simulink model "accelerate"  (R2022a)
settings: Solver=FixedStepDiscrete  StartTime=0.0  StopTime=inf  RelTol=1e-3  EnableMultiTasking=on
InitFcn:
  | run('busObjects.m')
model workspace (MAT data in the model file):
  omega = 8
  zeta = 0.05
undefined symbols (not defined in the file or in its folder): HS, IO291
libraries: aru_toolbox x6, eeGeneralControl x4, speedgoatlib_IO691 x3, speedgoatlib_IO291 x1
settings Model: SimulationMode=external  Creator=Mechatronics  LastModifiedBy=Mechatronics
settings SolverCC: ConcurrentTasks=on  AlgebraicLoopSolver=TrustRegion  PositivePriorityOrder=on  InsertRTBMode=Never (minimum delay)
settings DataIOCC: SaveFormat=Array  SaveState=on  SignalLoggingName=logsOut
settings OptimizationCC: BlockReduction=off  BooleanDataType=off  OptimizeBlockIOStorage=off  BufferReuse=off  GlobalBufferReuse=off  ExpressionFolding=off  LocalBlockOutputs=off  InitFltsAndDblsToZero=on  OptimizeDataStoreBuffers=off  BusAssignmentInplaceUpdate=off
settings DebuggingCC: SaveWithParameterizedLinksMsg=none  UnderspecifiedInitializationDetection=Classic  MergeDetectMultiDrivingBlocksExec=none  CheckExecutionContextPreStartOutputMsg=on  SignalResolutionControl=TryResolveAllWithWarning  TasksWithSamePriorityMsg=none  UnconnectedInputMsg=warning  UnconnectedOutputMsg=warning  UnconnectedLineMsg=warning  SFUnexpectedBacktrackingDiag=warning  SFNoUnconditionalDefaultTransitionDiag=warning  SFExecutionAtInitializationDiag=none  SFMachineParentedDataDiag=warning  ArithmeticOperatorsInVariantConditions=warning
settings HardwareCC: ProdBitPerLong=64  ProdLongLongMode=on  ProdHWDeviceType=Intel->x86-64 (Linux 64)
settings ModelReferenceCC: PropagateSignalLabelsOutOfModel=off
settings SFSimCC: SimUseLocalCustomCode=off  SimTargetLang=C++
settings RTWCC: Description=Simulink Real-Time  SystemTargetFile=slrealtime.tlc  TemplateMakefile=slrealtime_default_tmf  RTWUseLocalCustomCode=off  Toolchain=Simulink Real-Time Toolchain  BuildConfiguration=Faster Runs  CodeExecutionProfiling=on  TargetLang=C++  DLArmComputeVersion=19.05
settings CodeAppCC: StateflowObjectComments=on
settings SimulinkRealTimeTargetCC: MATLABClassNameForMDSCustomization=Simulink.SoftwareTarget.GRTCustomization  UseGCCFastMath=on
settings ConfigComp: CovMetricSettings=dw  CovSaveCumulativeToWorkspaceVar=on  CovSaveSingleToWorkspaceVar=on  CovExternalEMLEnable=off  CovSFcnEnable=off

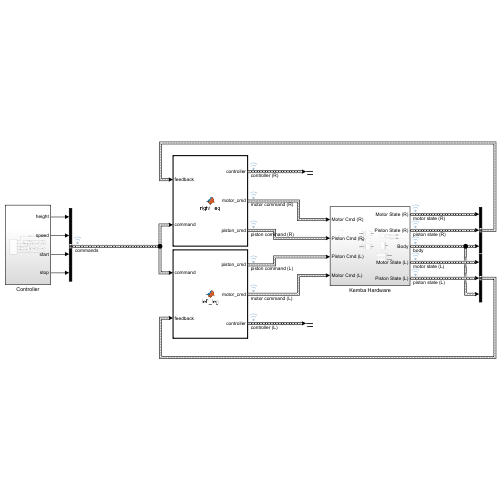
[thumbnail: Simulink's stored preview of the top-level diagram]
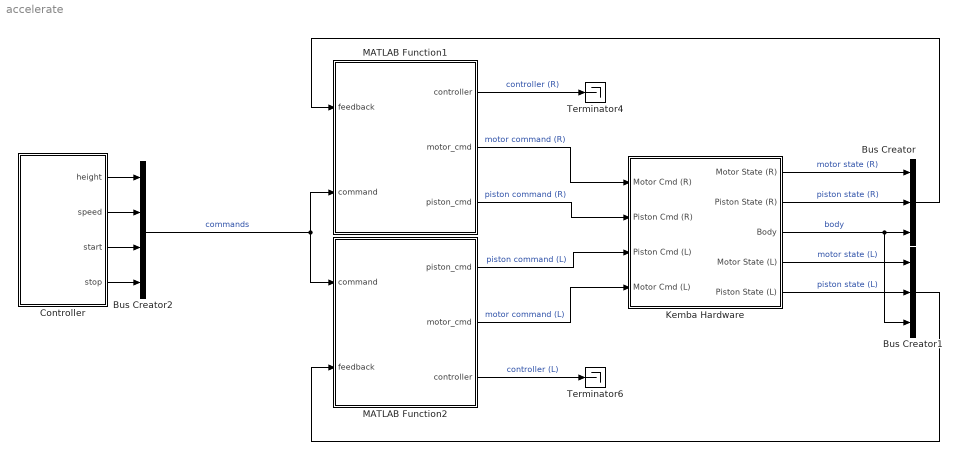
== system accelerate ==
  Bus Creator : BusCreator  Inputs=3  OutDataTypeStr=Bus: State  NonVirtualBus=on
      settings: InheritFromInputs=off
  Bus Creator1 : BusCreator  Inputs=3  OutDataTypeStr=Bus: State  NonVirtualBus=on
      settings: InheritFromInputs=off
  Bus Creator2 : BusCreator  Inputs=4  OutDataTypeStr=Bus: Command  NonVirtualBus=on
      settings: InheritFromInputs=off
  Controller : Subsystem
  Kemba Hardware : Subsystem
  MATLAB Function1 : MATLAB Function  TreatAsAtomicUnit=on  SystemSampleTime=0.001
  MATLAB Function2 : MATLAB Function  TreatAsAtomicUnit=on  SystemSampleTime=0.001
  Terminator4 : Terminator
  Terminator6 : Terminator
  wires:
  MATLAB Function1/3(piston_cmd) -> Kemba Hardware/2(Piston Cmd (R))  "piston command (R)"
  MATLAB Function2/1(piston_cmd) -> Kemba Hardware/3(Piston Cmd (L))  "piston command (L)"
  MATLAB Function1/2(motor_cmd) -> Kemba Hardware/1(Motor Cmd (R))  "motor command (R)"
  MATLAB Function2/2(motor_cmd) -> Kemba Hardware/4(Motor Cmd (L))  "motor command (L)"
  Kemba Hardware/4(Motor State (L)) -> Bus Creator1/1  "motor state (L)"
  Kemba Hardware/5(Piston State (L)) -> Bus Creator1/2  "piston state (L)"
  Kemba Hardware/3(Body) -> Bus Creator1/3, Bus Creator/3  "body"
  Kemba Hardware/2(Piston State (R)) -> Bus Creator/2  "piston state (R)"
  Kemba Hardware/1(Motor State (R)) -> Bus Creator/1  "motor state (R)"
  Bus Creator/1 -> MATLAB Function1/1(feedback)
  Bus Creator1/1 -> MATLAB Function2/2(feedback)
  Bus Creator2/1 -> MATLAB Function2/1(command), MATLAB Function1/2(command)  "commands"
  Controller/2(speed) -> Bus Creator2/2
  MATLAB Function1/1(controller) -> Terminator4/1  "controller (R)"
  MATLAB Function2/3(controller) -> Terminator6/1  "controller (L)"
  Controller/1(height) -> Bus Creator2/1
  Controller/3(start) -> Bus Creator2/3
  Controller/4(stop) -> Bus Creator2/4

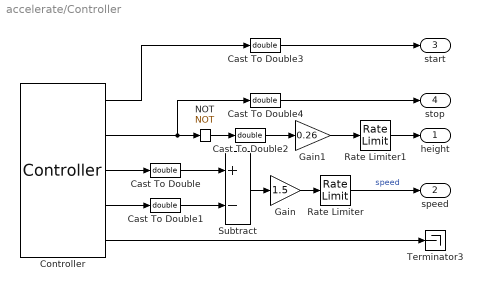
== system accelerate/Controller ==
  Cast To Double{,1..4} (5 alike) : DataTypeConversion  OutDataTypeStr=double  SaturateOnIntegerOverflow=off  RndMeth=Floor
  Controller : aru_toolbox/Controller
      link override "LVTTL digital input ": parInternalModuleId=1
      settings: SourceProductName=ARU Toolbox
  Gain : Gain  Gain=1.5
  Gain1 : Gain  Gain=0.26
  NOT : Logic  Operator=NOT  IconShape=distinctive  AllPortsSameDT=off  OutDataTypeStr=boolean
  Rate Limiter : RateLimiter  RisingSlewLimit=0.3  FallingSlewLimit=-0.3  SampleTimeMode=inherited
  Rate Limiter1 : RateLimiter  RisingSlewLimit=0.05  FallingSlewLimit=-0.05  SampleTimeMode=inherited  InitialCondition=0.26
  Subtract : Sum  Inputs=+-
  Terminator3 : Terminator
  height : Outport
  speed : Outport  Port=2
  start : Outport  Port=3
  stop : Outport  Port=4
  wires:
  Gain1/1 -> Rate Limiter1/1
  Rate Limiter/1 -> speed/1  "speed"
  Subtract/1 -> Gain/1
  Controller/5 -> Terminator3/1
  Controller/2 -> Cast To Double4/1, NOT/1
  Controller/3 -> Cast To Double/1
  Gain/1 -> Rate Limiter/1
  Controller/4 -> Cast To Double1/1
  Cast To Double/1 -> Subtract/1
  Cast To Double1/1 -> Subtract/2
  Controller/1 -> Cast To Double3/1
  Rate Limiter1/1 -> height/1
  Cast To Double3/1 -> start/1
  NOT/1 -> Cast To Double2/1
  Cast To Double2/1 -> Gain1/1
  Cast To Double4/1 -> stop/1

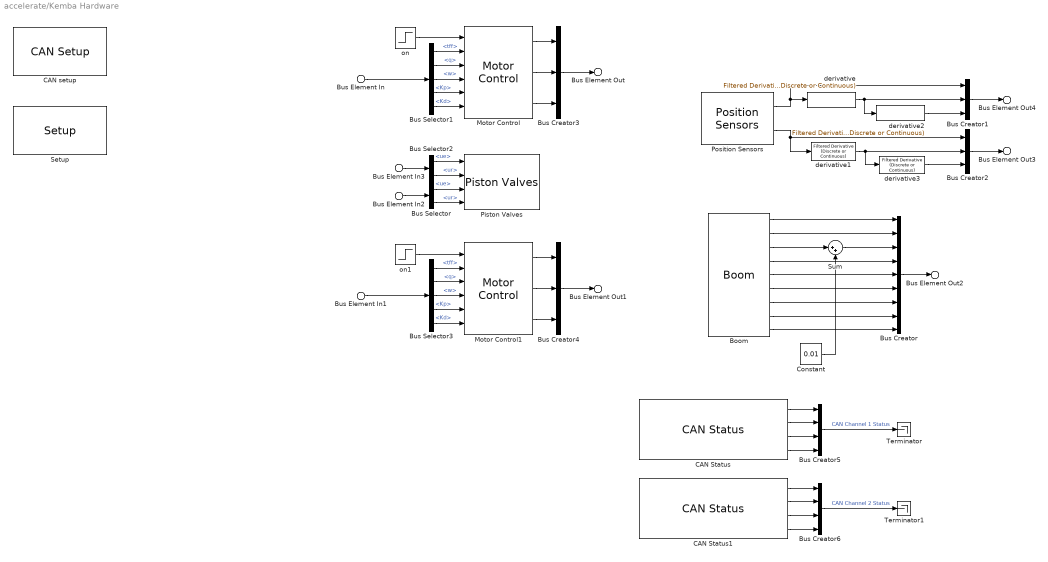
== system accelerate/Kemba Hardware ==
  Bus Element In : Inport  PortName=Motor Cmd (R)
  Bus Element In2 : Inport  Port=2  PortName=Piston Cmd (R)
  Bus Element In3 : Inport  Port=3  PortName=Piston Cmd (L)
  Bus Element In1 : Inport  Port=4  PortName=Motor Cmd (L)
  Boom : aru_toolbox/Boom  ts=0.001
      link override Serial Read HW FIFO: pciSlot=-1  board=IO393-50k
      link override Serial Setup: pciSlot=-1  board=IO393-50k
      settings: SourceProductName=ARU Toolbox
  Bus Creator : BusCreator  Inputs=9  OutDataTypeStr=Bus: BodyState  NonVirtualBus=on
      settings: InheritFromInputs=off
  Bus Creator1 : BusCreator  Inputs=3  OutDataTypeStr=Bus: PistonState  NonVirtualBus=on
      settings: InheritFromInputs=off
  Bus Creator2 : BusCreator  Inputs=3  OutDataTypeStr=Bus: PistonState  NonVirtualBus=on
      settings: InheritFromInputs=off
  Bus Creator3 : BusCreator  Inputs=3  OutDataTypeStr=Bus: MotorState  NonVirtualBus=on
      settings: InheritFromInputs=off
  Bus Creator4 : BusCreator  Inputs=3  OutDataTypeStr=Bus: MotorState  NonVirtualBus=on
      settings: InheritFromInputs=off
  Bus Creator5 : BusCreator  Inputs=4  OutDataTypeStr=Bus: CAN  NonVirtualBus=on
      settings: InheritFromInputs=off
  Bus Creator6 : BusCreator  Inputs=4  OutDataTypeStr=Bus: CAN  NonVirtualBus=on
      settings: InheritFromInputs=off
  Bus Selector : BusSelector  OutputSignals=ue,ur
  Bus Selector1 : BusSelector  OutputSignals=tff,q,w,Kp,Kd
  Bus Selector2 : BusSelector  OutputSignals=ue,ur
  Bus Selector3 : BusSelector  OutputSignals=tff,q,w,Kp,Kd
  CAN Status : speedgoatlib_IO691/Legacy/CAN Status  moduleId=1  sampleTime=0.001  channel=1  busRecovery=Auto  arrayOutput=off  controllerCpuLoad=off  controllerLiveCount=off  initModeAct=off  avgBusLoad=on  receiving=off  RxQueueEmpty=off  dataOverrunRcv=off  rxBufferLevel=off  txPending=off  dataOverrunTx=off  txBufferLevel=off  errWarnLimit=on  errPassLimit=on  errBusOff=on  busRecoveryCounter=off  busCouplingErr=off  transceiverErr=off  opMode=off  brp=off  timeSegment1=off  timeSegment2=off  synchronisationJumpWidth=off  dataTSEG1=off  dataTSEG2=off  dataSJW=off  moduleType=691  qtyStatBlk=1  ptIdx=0  isFDMod=0
      settings: SourceProductName=Simulink Real-Time: Speedgoat I/O Blockset
  CAN Status1 : speedgoatlib_IO691/Legacy/CAN Status  moduleId=1  sampleTime=0.001  channel=2  busRecovery=Auto  arrayOutput=off  controllerCpuLoad=off  controllerLiveCount=off  initModeAct=off  avgBusLoad=on  receiving=off  RxQueueEmpty=off  dataOverrunRcv=off  rxBufferLevel=off  txPending=off  dataOverrunTx=off  txBufferLevel=off  errWarnLimit=on  errPassLimit=on  errBusOff=on  busRecoveryCounter=off  busCouplingErr=off  transceiverErr=off  opMode=off  brp=off  timeSegment1=off  timeSegment2=off  synchronisationJumpWidth=off  dataTSEG1=off  dataTSEG2=off  dataSJW=off  moduleType=691  qtyStatBlk=1  ptIdx=0  isFDMod=0
      settings: SourceProductName=Simulink Real-Time: Speedgoat I/O Blockset
  CAN setup : speedgoatlib_IO691/Legacy/CAN Setup   moduletype=IO691  id=1  pciSlot=-1  chn1=CAN (HS)  chn2=CAN (HS)  chn3=Disabled  chn4=Disabled  initStruct=[]  termStruct=[struct('Channel',1,'Protocol','CAN','BRS',0,'Type','Standard','Identifier',1,'Data',[255, 255, 255, 255, 255, 255, 255, 253],'Pause',0.001), struct('Channel',2,'Protocol','CAN','BRS',0,'Type','Standard','Identifier',2,'Data',[255, 255, 255, 255, 255, 255, 255, 253],'Pause',0.001)]  ArbitrationbdrChn1=1.0 MBaud  ArbitrationManbdrChn1=[2,8,31,8]  FdbdrChn1=1.0 MBaud  FdManbdrChn1=[2,8,31,8]  ArbitrationbdrChn2=1.0 MBaud  ArbitrationManbdrChn2=[2,8,31,8]  FdbdrChn2=1.0 MBaud  FdManbdrChn2=[2,8,31,8]  ArbitrationbdrChn3=1.0 MBaud  ArbitrationManbdrChn3=[2,8,31,8]  FdbdrChn3=5.0 MBaud  FdManbdrChn3=[2,2,5,2]  ArbitrationbdrChn4=1.0 MBaud  ArbitrationManbdrChn4=[2,8,31,8]  FdbdrChn4=5.0 MBaud  FdManbdrChn4=[2,2,5,2]  moduleInitValues=[691 1 -1 -1]
      settings: SourceProductName=Simulink Real-Time: Speedgoat I/O Blockset
  Constant : Constant  Value=0.01
  Motor Control : aru_toolbox/Motor Control  id=1  channel=1  offset=0.8494-pi
      settings: SourceProductName=ARU Toolbox
  Motor Control1 : aru_toolbox/Motor Control  id=2  channel=2  offset=-0.5243
      settings: SourceProductName=ARU Toolbox
  Piston Valves : aru_toolbox/Piston Valves  SystemSampleTime=-1  VariantActivationTime=update diagram  Latency=0  AutoFrameSizeCalculation=off
      settings: SourceProductName=ARU Toolbox
  Position Sensors : aru_toolbox/Position Sensors  stroke1=0.07  stroke2=0.07
      settings: SourceProductName=ARU Toolbox
  "Setup " : speedgoatlib_IO291/Setup   parInternalModuleId=1  parPciSlot=-1  parModuleId=1  parModuleType=IO291-HS  parTtlDoChannels=[]  parTtlDoInitValues=1  parTtlDoReset=1  parTtlDiChannels=[1 2 3 4 5]  parIsolDiChannels=[]  parFetDoChannels=[1 2 3 4]  parFetDoInitValues=0  parFetDoReset=1
      settings: SourceProductName=Simulink Real-Time: Speedgoat I/O Blockset
  Sum : Sum  Inputs=|++
  Terminator : Terminator
  Terminator1 : Terminator
  derivative{,1..3} (4 alike) : eeGeneralControl/Filtered Derivative (Discrete or Continuous)  K=1  T=0.002  B=inf  A=-inf  minRatio=2  init_option=Inherited from block input  x0=0  Ts=0.001
      settings: SourceProductBaseCode=PS
  on : Step  SampleTime=0
  on1 : Step  Time=2  SampleTime=0
  Bus Element Out : Outport  PortName=Motor State (R)
  Bus Element Out4 : Outport  Port=2  PortName=Piston State (R)
  Bus Element Out2 : Outport  Port=3  PortName=Body
  Bus Element Out1 : Outport  Port=4  PortName=Motor State (L)
  Bus Element Out3 : Outport  Port=5  PortName=Piston State (L)
  wires:
  Bus Selector3/4 -> Motor Control1/5  "<Kp>"
  on1/1 -> Motor Control1/1
  Motor Control1/3 -> Bus Creator4/3
  Bus Selector1/3 -> Motor Control/4  "<w>"
  Bus Selector3/2 -> Motor Control1/3  "<q>"
  Bus Selector1/4 -> Motor Control/5  "<Kp>"
  Bus Selector3/3 -> Motor Control1/4  "<w>"
  on/1 -> Motor Control/1
  Motor Control/2 -> Bus Creator3/2
  Motor Control1/1 -> Bus Creator4/1
  Bus Selector1/1 -> Motor Control/2  "<tff>"
  Bus Selector1/2 -> Motor Control/3  "<q>"
  Bus Selector3/1 -> Motor Control1/2  "<tff>"
  Bus Selector3/5 -> Motor Control1/6  "<Kd>"
  Bus Selector1/5 -> Motor Control/6  "<Kd>"
  Motor Control1/2 -> Bus Creator4/2
  Motor Control/1 -> Bus Creator3/1
  Motor Control/3 -> Bus Creator3/3
  Bus Element In/1 -> Bus Selector1/1
  Bus Element In1/1 -> Bus Selector3/1
  Bus Creator3/1 -> Bus Element Out/1
  Bus Creator4/1 -> Bus Element Out1/1
  derivative/1 -> derivative2/1, Bus Creator1/2
  Position Sensors/1 -> Bus Creator1/1, derivative/1
  derivative1/1 -> derivative3/1, Bus Creator2/2
  Position Sensors/2 -> derivative1/1, Bus Creator2/1
  Boom/3 -> Sum/1
  Boom/9 -> Bus Creator/9
  Boom/4 -> Bus Creator/4
  Boom/5 -> Bus Creator/5
  Boom/7 -> Bus Creator/7
  Boom/6 -> Bus Creator/6
  Boom/8 -> Bus Creator/8
  Boom/1 -> Bus Creator/1
  Boom/2 -> Bus Creator/2
  Bus Element In2/1 -> Bus Selector/1
  Bus Element In3/1 -> Bus Selector2/1
  Bus Creator/1 -> Bus Element Out2/1
  Bus Creator1/1 -> Bus Element Out4/1
  Bus Creator2/1 -> Bus Element Out3/1
  Bus Selector2/1 -> Piston Valves/1  "<ue>"
  Bus Selector2/2 -> Piston Valves/2  "<ur>"
  Bus Selector/1 -> Piston Valves/3  "<ue>"
  Bus Selector/2 -> Piston Valves/4  "<ur>"
  derivative2/1 -> Bus Creator1/3
  derivative3/1 -> Bus Creator2/3
  CAN Status1/4 -> Bus Creator6/4
  CAN Status1/3 -> Bus Creator6/3
  Bus Creator6/1 -> Terminator1/1  "CAN Channel 2 Status"
  Bus Creator5/1 -> Terminator/1  "CAN Channel 1 Status"
  CAN Status/4 -> Bus Creator5/4
  CAN Status1/1 -> Bus Creator6/1
  CAN Status/3 -> Bus Creator5/3
  CAN Status1/2 -> Bus Creator6/2
  CAN Status/2 -> Bus Creator5/2
  CAN Status/1 -> Bus Creator5/1
  Sum/1 -> Bus Creator/3
  Constant/1 -> Sum/2

== matlab function accelerate/MATLAB Function2 ==
  data: command input Bus: Command; feedback input Bus: State; piston_cmd output Bus: PistonCmd; motor_cmd output Bus: MotorCmd; controller output Bus: Controller
function [piston_cmd, motor_cmd, controller] = left_leg(command, feedback) %#codegen

% initialisation
hip.y = 0; hip.dy = 0; hip.y_min = 0; hip.y_max = 0;
foot.y = 0; foot.height = 0; foot.contact = false; foot.radius = 20e-3;

% constants
contact_threshold = 1e-2; % m foot radius
contact_acceleration_threshold = -100; % m/s^2
retract_duration = 17; % 17ms
hip.amplitude = 0.01;
hip.y_min = command.height - 0.5*hip.amplitude;
hip.y_max = command.height + 0.5*hip.amplitude;

motor = feedback.Motor;
piston = feedback.Piston;
body = feedback.Body;

% kinematics
[r,dr,phi,~] = virtural_leg_b(piston.v, body.dr, motor.w, piston.p, body.r, motor.q);
[~, ~ ,hip.y, hip.dy] = hip_pos_b(body.dr, body.dx, body.dy, body.r, body.x, body.y);
[~,foot.y] = foot_pos_b(piston.p, body.r, motor.q, body.x, body.y);

persistent state
persistent retract_timer
persistent ground_offset
persistent Ts
if isempty(state)
    state = States.Rest;
end
if isempty(retract_timer)
    retract_timer = 0;
end
if isempty(ground_offset)
    ground_offset = 0;
end
if isempty(Ts)
    Ts = 0;
end

% contact detection
foot.height = foot.y + ground_offset;
if foot.height > contact_threshold
    foot.contact = false;
else
    foot.contact = true;
end

% state transitions
switch(state)
    case States.Rest
        if (body.r > 0.1) && (body.dr < 1.0) && (command.start) % wait until right leg has pushed off a bit
            state = States.Stance;
            ground_offset = -foot.y;
        end
    case States.Flight
        if ((hip.y + ground_offset) < ((2.5*hip.dy*hip.dy)/(2*50) + hip.y_min)) && (hip.dy < 0)
            state = States.Loading;
        elseif (hip.y_min < 0.17) && (command.stop)
            state = States.Rest;
        end
    case States.Loading
        if (piston.a < contact_acceleration_threshold) || (foot.contact)
            Ts = 0;
            state = States.Stance;
        end
    case States.Stance
        if hip.dy > 0
            if (hip.y + ground_offset) > ((hip.dy*hip.dy)/(-2*9.81) + hip.y_max)
                retract_timer = 0;
                ground_offset = -foot.y; % update ground offset
                state = States.Unloading;
            end
        end
    case States.Unloading
        if ~foot.contact
            state = States.Flight;
        end
end


% control piston
switch(state)
    case {States.Loading, States.Stance}
        piston_cmd.ue = 1;
        piston_cmd.ur = 0;
    case States.Unloading
        piston_cmd.ue = 0;
        if retract_timer < retract_duration
            piston_cmd.ur = 1;
        else
            piston_cmd.ur = 0;
        end
        retract_timer = retract_timer + 1;
    otherwise
        piston_cmd.ue = 0;
        piston_cmd.ur = 0;
end

% stance timer
switch(state)
    case {States.Stance, States.Unloading}
        Ts = Ts + 0.001;
end

% control motor
switch(state)
    case {States.Stance, States.Unloading, States.Loading}
        phi_d = -pi/2;
        dphi_d = (dr*cos(phi) + command.speed)/(r*sin(phi));
        Kp = 0;
        Kd = 4;
    case {States.Flight}
        foot_offset = (body.dx*(0.1))/(2*r);
        foot_offset = max(min(foot_offset,1),-1);
        phi_d = -pi/2 + asin(foot_offset);
        dphi_d = 0;
        Kp = 100; % 80
        Kd = 4;
    case States.Rest
        foot_offset = (command.speed*(0.08))/(2*r);
        foot_offset = max(min(foot_offset,1),-1);
        phi_d = -pi/2 + asin(foot_offset);
        dphi_d = 0;
        Kp = 50;
        Kd = 4;
    otherwise
        phi_d = -pi/2;
        dphi_d = 0;
        Kp = 50;
        Kd = 4;
end
 
[theta_m_des,dtheta_m_des] = phi_tracking_b(piston.v, dphi_d, body.dr, piston.p, phi_d, body.r);
% bound motor angle to not break pneumatics
theta_m_des =  min(theta_m_des, 0);

motor_cmd.q = theta_m_des;
motor_cmd.w = dtheta_m_des;
motor_cmd.Kp = Kp;
motor_cmd.Kd = Kd;
motor_cmd.tff = 0;

controller.state = state;
controller.Ts = Ts;
 
end

== matlab function accelerate/MATLAB Function1 ==
  data: feedback input Bus: State; controller output Bus: Controller; motor_cmd output Bus: MotorCmd; piston_cmd output Bus: PistonCmd; command input Bus: Command
function [controller, motor_cmd, piston_cmd] = right_leg(feedback, command) %#codegen

% initialisation
hip.y = 0; hip.dy = 0; hip.y_min = 0; hip.y_max = 0;
foot.y = 0; foot.height = 0; foot.contact = false; foot.radius = 20e-3;

motor = feedback.Motor;
piston = feedback.Piston;
body = feedback.Body;

% kinematics
[r,dr,phi,~] = virtural_leg_f(piston.v, body.dr, motor.w, piston.p, body.r, motor.q);
[~, ~ ,hip.y, hip.dy] = hip_pos_f(body.dr, body.dx, body.dy, body.r, body.x, body.y);
[~,foot.y] = foot_pos_f(piston.p, body.r, motor.q, body.x, body.y);

% constants
contact_threshold = 1e-2; % m relies on ground being flat
contact_acceleration_threshold = -100; % m/s^2
retract_duration = 17; % 17ms
hip.amplitude = 0.01;
hip.y_min = command.height - 0.5*hip.amplitude;
hip.y_max = command.height + 0.5*hip.amplitude;

persistent state
persistent retract_timer
persistent ground_offset
persistent Ts
if isempty(state)
    state = States.Rest;
end
if isempty(retract_timer)
    retract_timer = 0;
end
if isempty(ground_offset)
    ground_offset = 0;
end
if isempty(Ts)
    Ts = 0;
end
 
% contact detection
foot.height = foot.y + ground_offset;
if foot.height > contact_threshold
    foot.contact = false;
else
    foot.contact = true;
end
 
% state transitions
switch(state)
    case States.Rest
        if command.start
            state = States.Accelerate;
            ground_offset = -foot.y;
        end
    case States.Accelerate
        if hip.dy > 0
            if (hip.y + ground_offset) > ((hip.dy*hip.dy)/(-2*9.81) + hip.y_max + 0.02)
                retract_timer = 0;
                ground_offset = -foot.y;
                state = States.Unloading;
            end
        end
    case States.Flight
        if ((hip.y + ground_offset) < ((2.5*hip.dy*hip.dy)/(2*50) + hip.y_min)) && (hip.dy < 0)
            state = States.Loading;
        elseif (hip.y_min < 0.17) && (command.stop)
            state = States.Rest;
        end
    case States.Loading
        if (piston.a < contact_acceleration_threshold) || (foot.contact)
            Ts = 0;
            state = States.Stance;
        end
    case States.Stance
        if hip.dy > 0
            if (hip.y + ground_offset) > ((hip.dy*hip.dy)/(-2*9.81) + hip.y_max)
                retract_timer = 0;
                ground_offset = -foot.y; % update ground offset
                state = States.Unloading;
            end
        end
    case States.Unloading
        if ~foot.contact
            state = States.Flight;
        end
end
 
 
% control piston
switch(state)
    case {States.Loading, States.Stance, States.Accelerate}
        piston_cmd.ue = 1;
        piston_cmd.ur = 0;
    case States.Unloading
        piston_cmd.ue = 0;
        if retract_timer < retract_duration
            piston_cmd.ur = 1;
        else
            piston_cmd.ur = 0;
        end
        retract_timer = retract_timer + 1;
    otherwise
        piston_cmd.ue = 0;
        piston_cmd.ur = 0;
end

% stance timer
switch(state)
    case {States.Stance, States.Unloading}
        Ts = Ts + 0.001;
end
 
% control motor
switch(state)
    case {States.Stance, States.Unloading, States.Loading}
        phi_d = -pi/2;
        dphi_d = (dr*cos(phi) + command.speed)/(r*sin(phi));
        Kp = 0;
        Kd = 4;
    case States.Accelerate
        phi_d = -pi/2;
        dphi_d = 0;
        Kp = 100;
        Kd = 4;
    case {States.Flight}
        foot_offset = (body.dx*(0.1))/(2*r);
        foot_offset = max(min(foot_offset,1),-1);
        phi_d = -pi/2 + asin(foot_offset);
        dphi_d = 0;
        Kp = 100; % 80
        Kd = 4; % 2
    otherwise
        phi_d = -pi/2;
        dphi_d = 0;
        Kp = 50;
        Kd = 4;
end

[theta_m_des, dtheta_m_des] = phi_tracking_f(piston.v, dphi_d, body.dr, piston.p, phi_d, body.r);
% bound motor angle to not break pneumatics
theta_m_des = max(-pi, theta_m_des);

motor_cmd.q = theta_m_des;
motor_cmd.w = dtheta_m_des;
motor_cmd.Kp = Kp;
motor_cmd.Kd = Kd;
motor_cmd.tff = 0;

controller.state = state;
controller.Ts = Ts;
 
end
